simulink model "Flight_Model_2020b_11_28_2020"  (R2021a)
settings: Solver=ode45  StartTime=0.0  StopTime=100  RelTol=1e-3  EnableMultiTasking=on
model workspace (MAT data in the model file):
  bodyLength = 5
  brakesCd = 1
  brakesOn = 1
  dryCG = 1.9
  dryMass = 23
  finArea = 0.2
  finChordAngle = 0.5236
  finSpan = 0.4
  fullBrakesOn = 0
  gravity = 9.8067
  noseLength = 0.5
  propMass = 7.183
  refArea = 0.0182
  rocketCP = 1
  rocketDiam = 0.197
  targetAlt = 3048
  thrust = [0; 2638.366; 2528.97; 3063.078; 2426.009; 2548.275; 2599.755; 2554.71; 2644.801; 2638.366; 2561.145; 2606.19; 2638.366; 2638.366; 2580.45; 2496.795; 2335.919; 2213.653; 2129.998; 1653.805; 888.035; 630.634; 450.453; 289.577; 135.136; 25.74; 0]
  time = [0; 0.045; 0.067; 0.084; 0.124; 0.186; 0.231; 0.298; 0.371; 0.534; 0.979; 1.142; 2.002; 2.289; 2.761; 3.121; 3.436; 3.678; 3.79; 4.004; 4.415; 4.538; 4.656; 4.82; 5.005; 5.219; 5.371]
  totalImpulse = 10831
  vehicleCd = 0.8
  wetCG = 2.1
  wetMass = 30
undefined symbols (not defined in the file): Earth, WGS84, X, Y, Z
libraries: sm_lib x19, nesl_utility x10, aerolibasang x4, commchan3 x3, aerolibbdyn x2, aerolibwind2 x2, shared6dof x2, simulink x2, aerolibtransform2 x1, aerolibfltsims x1, aerolibatmos2 x1, aerolibconvert2 x1
(part 1 of 2)
settings Model: Creator=jacob  LastModifiedBy=alhus
settings SolverCC: AlgebraicLoopSolver=TrustRegion
settings DataIOCC: LimitDataPoints=on  SaveFormat=Array  ReturnWorkspaceOutputs=off
settings OptimizationCC: LifeSpan=inf
settings DebuggingCC: SFUnexpectedBacktrackingDiag=warning  SFNoUnconditionalDefaultTransitionDiag=warning  SFExecutionAtInitializationDiag=none  SFMachineParentedDataDiag=warning  ArithmeticOperatorsInVariantConditions=warning
settings HardwareCC: ProdBitPerPointer=32  ProdBitPerSizeT=32  ProdBitPerPtrDiffT=32  ProdLargestAtomicFloat=None  ProdIntDivRoundTo=Undefined  ProdEndianess=Unspecified  ProdWordSize=32  ProdHWDeviceType=32-bit Generic
settings ModelReferenceCC: PropagateSignalLabelsOutOfModel=off
settings SFSimCC: SimUseLocalCustomCode=off  CustomCodeUndefinedFunction=UseInterfaceOnly
settings RTWCC: RTWUseLocalCustomCode=off
settings CodeAppCC: StateflowObjectComments=on
settings GRTTargetCC: TargetLangStandard=C89/C90 (ANSI)
settings ConfigComp: CovMetricSettings=dw  CovSaveCumulativeToWorkspaceVar=on  CovSaveSingleToWorkspaceVar=on  CovExternalEMLEnable=off
settings SimscapeCC: SimscapeNormalizeSystem=off
settings ConfigurationSet: Description=SimMechanics 2G

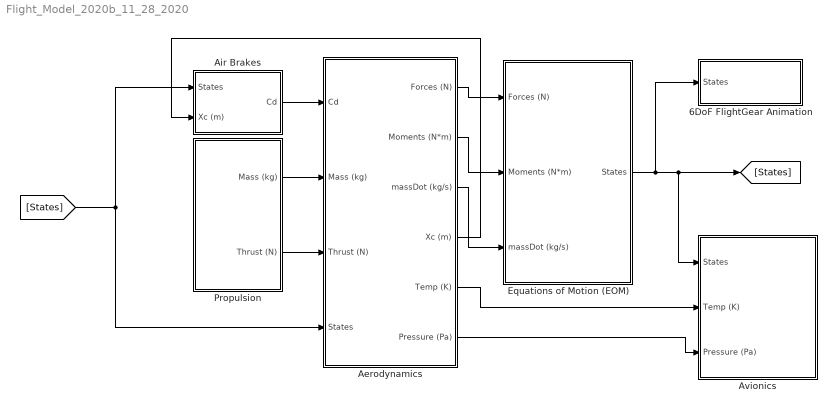
== system Flight_Model_2020b_11_28_2020 ==
  6DoF FlightGear Animation : Subsystem
  Aerodynamics : Subsystem
  Air Brakes : Subsystem
  Avionics : Subsystem
  Equations of Motion (EOM) : Subsystem
  Propulsion : Subsystem
  wires:
  Aerodynamics/1(Forces (N)) -> Equations of Motion (EOM)/1(Forces (N))
  Aerodynamics/2(Moments (N*m)) -> Equations of Motion (EOM)/2(Moments (N*m))
  Propulsion/1(Mass (kg)) -> Aerodynamics/2(Mass (kg))
  Propulsion/2(Thrust (N)) -> Aerodynamics/3(Thrust (N))
  Air Brakes/1("Cd ") -> Aerodynamics/1(Cd)
  Equations of Motion (EOM)/1(States) -> Avionics/1(States), [States], 6DoF FlightGear Animation/1(States)
  [States] -> Air Brakes/1(States), Aerodynamics/4(States)
  Aerodynamics/3(massDot (kg/s)) -> Equations of Motion (EOM)/3(massDot (kg/s))
  Aerodynamics/4(Xc (m)) -> Air Brakes/2(Xc (m))
  Aerodynamics/5(Temp (K)) -> Avionics/2(Temp (K))
  Aerodynamics/6(Pressure (Pa)) -> Avionics/3(Pressure (Pa))

== system Flight_Model_2020b_11_28_2020/6DoF FlightGear Animation ==
  States : Inport
  Bus Selector : BusSelector  OutputSignals=signal2,signal3
  Constant : Constant  Value=0
  Demux : Demux  Outputs=2
  Demux1 : Demux  Outputs=3
  Display : Display
  Display1 : Display
  Display2 : Display
  Flat Earth to LLA : aerolibtransform2/Flat Earth to LLA  units=Metric (MKS)  ptype=Earth (WGS84)  F=1/298.257223563  R=6378137  refPosPort=off  LL0=[0 10]  psi=0
  FlightGear Preconfigured 6DoF Animation : aerolibfltsims/FlightGear Preconfigured 6DoF Animation  xFlightGearVersion=v3.0  DestinationIpAddress=127.0.0.1  DestinationPort=5502  SampleTime=1/30  packetVersion=24
  Mux : Mux  Inputs=6
  wires:
  States/1 -> Bus Selector/1
  Constant/1 -> Flat Earth to LLA/2
  Mux/1 -> FlightGear Preconfigured 6DoF Animation/1
  Flat Earth to LLA/1 -> Demux/1
  Demux/1 -> Display1/1, Mux/2
  Demux/2 -> Display2/1, Mux/1
  Flat Earth to LLA/2 -> Display/1, Mux/3
  Demux1/2 -> Mux/5
  Demux1/3 -> Mux/6
  Demux1/1 -> Mux/4
  Bus Selector/1 -> Flat Earth to LLA/1  "<signal2>"
  Bus Selector/2 -> Demux1/1  "<signal3>"

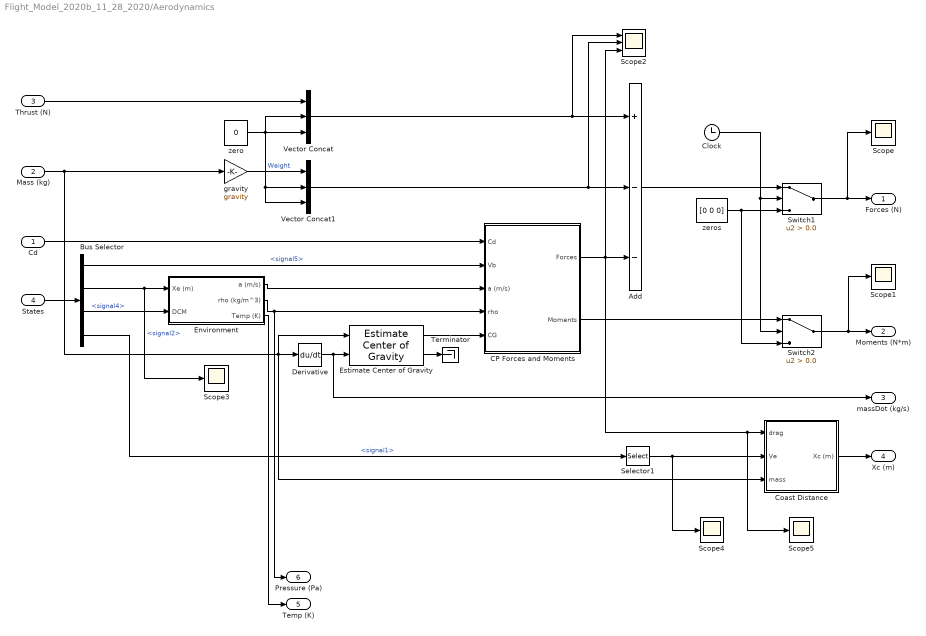
== system Flight_Model_2020b_11_28_2020/Aerodynamics ==
  Cd : Inport
  Mass (kg) : Inport  Port=2
  Thrust (N) : Inport  Port=3
  States : Inport  Port=4
  Add : Sum  Inputs=+--
  Bus Selector : BusSelector  OutputSignals=signal5,signal2,signal4,signal1
  CP Forces and Moments : Subsystem
  Clock : Clock
  Coast Distance : Subsystem
  Derivative : Derivative
  Environment : Subsystem
  Estimate Center of Gravity : aerolibbdyn/Estimate Center of Gravity  fmass=wetMass  emass=dryMass  fcg=[wetCG 0 0]'  ecg=[dryCG 0 0]'
      settings: SourceProductBaseCode=AE
  Scope{,1,3..5} (5 alike) : Scope
  Scope2 : Scope  NumInputPorts=3
  Selector1 : Selector  InputPortWidth=3  IndexOptions=Index vector (dialog)  Indices=1  OutputSizes=1
  Switch1 : Switch  Criteria=u2 > Threshold  Threshold=0.0
  Switch2 : Switch  Criteria=u2 > Threshold  Threshold=0.0
  Terminator : Terminator
  Vector Concat : Concatenate  NumInputs=3
  Vector Concat1 : Concatenate  NumInputs=3
  gravity : Gain  Gain=gravity
  "zero " : Constant  Value=0
  "zeros " : Constant  Value=[0 0 0]
  Forces (N) : Outport
  Moments (N*m) : Outport  Port=2
  massDot (kg/s) : Outport  Port=3
  Xc (m) : Outport  Port=4
  Temp (K) : Outport  Port=5
  Pressure (Pa) : Outport  Port=6
  wires:
  Mass (kg)/1 -> Coast Distance/3(mass), Estimate Center of Gravity/1, Derivative/1, gravity/1
  Derivative/1 -> Estimate Center of Gravity/2, massDot (kg/s)/1
  Estimate Center of Gravity/2 -> Terminator/1
  Estimate Center of Gravity/1 -> CP Forces and Moments/5(CG)
  Cd/1 -> CP Forces and Moments/1(Cd)
  Environment/2(rho (kg/m^3)) -> Pressure (Pa)/1, CP Forces and Moments/4(rho)
  Add/1 -> Switch1/1
  Switch1/1 -> Scope/1, Forces (N)/1
  "zeros "/1 -> Switch2/3, Switch1/3
  Clock/1 -> Switch2/2, Switch1/2
  Switch2/1 -> Scope1/1, Moments (N*m)/1
  States/1 -> Bus Selector/1
  Environment/1(a (m/s)) -> CP Forces and Moments/3(a (m/s))
  Bus Selector/1 -> CP Forces and Moments/2(Vb)  "<signal5>"
  Bus Selector/2 -> Environment/1(Xe (m)), Scope3/1  "<signal2>"
  Bus Selector/3 -> Environment/2(DCM)  "<signal4>"
  "zero "/1 -> Vector Concat/2, Vector Concat/3, Vector Concat1/2, Vector Concat1/3
  Thrust (N)/1 -> Vector Concat/1
  Vector Concat/1 -> Scope2/1, Add/1
  Vector Concat1/1 -> Scope2/2, Add/2
  CP Forces and Moments/2(Moments) -> Switch2/1
  gravity/1 -> Vector Concat1/1  "Weight"
  CP Forces and Moments/1(Forces) -> Scope5/1, Coast Distance/1(drag), Add/3, Scope2/3
  Bus Selector/4 -> Selector1/1  "<signal1>"
  Coast Distance/1(Xc (m)) -> Xc (m)/1
  Selector1/1 -> Coast Distance/2(Ve), Scope4/1
  Environment/3(Temp (K)) -> Temp (K)/1

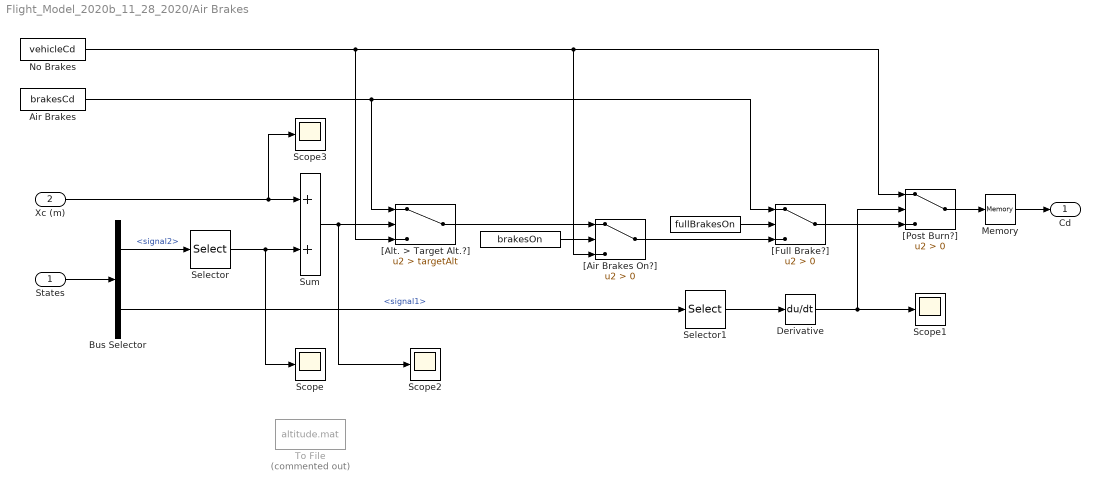
== system Flight_Model_2020b_11_28_2020/Air Brakes ==
  States : Inport
  Xc (m) : Inport  Port=2
  " " : Constant  Value=fullBrakesOn
  "  " : Constant  Value=brakesOn
  Air Brakes : Constant  Value=brakesCd
  Bus Selector : BusSelector  OutputSignals=signal2,signal1
  Derivative : Derivative
  Memory : Memory
  No Brakes : Constant  Value=vehicleCd
  Scope{,1..3} (4 alike) : Scope
  "Selector " : Selector  InputPortWidth=3  IndexOptions=Index vector (dialog)  Indices=1  OutputSizes=1
  Selector1 : Selector  InputPortWidth=3  IndexOptions=Index vector (dialog)  Indices=1  OutputSizes=1
  Sum : Sum
  To File : ToFile  Commented=on  Filename=altitude.mat  SaveFormat=Timeseries
  "[Air Brakes On?]" : Switch  Description=[Air Brakes On?]  Criteria=u2 > Threshold
  "[Alt. > Target Alt.?]" : Switch  Criteria=u2 > Threshold  Threshold=targetAlt
  "[Full Brake?]" : Switch  Criteria=u2 > Threshold
  "[Post Burn?]" : Switch  Criteria=u2 > Threshold
  "Cd " : Outport
  wires:
  Sum/1 -> Scope2/1, "[Alt. > Target Alt.?]"/2
  "[Post Burn?]"/1 -> Memory/1
  No Brakes/1 -> "[Alt. > Target Alt.?]"/3, "[Post Burn?]"/1, "[Air Brakes On?]"/3
  " "/1 -> "[Full Brake?]"/2
  Air Brakes/1 -> "[Alt. > Target Alt.?]"/1, "[Full Brake?]"/1
  "[Full Brake?]"/1 -> "[Post Burn?]"/3
  "Selector "/1 -> Scope/1, Sum/2
  "  "/1 -> "[Air Brakes On?]"/2
  "[Air Brakes On?]"/1 -> "[Full Brake?]"/3
  "[Alt. > Target Alt.?]"/1 -> "[Air Brakes On?]"/1
  States/1 -> Bus Selector/1
  Selector1/1 -> Derivative/1
  Derivative/1 -> "[Post Burn?]"/2, Scope1/1
  Bus Selector/1 -> "Selector "/1  "<signal2>"
  Xc (m)/1 -> Scope3/1, Sum/1
  Bus Selector/2 -> Selector1/1  "<signal1>"
  Memory/1 -> "Cd "/1

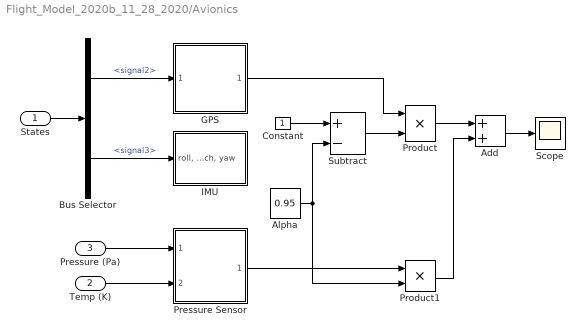
== system Flight_Model_2020b_11_28_2020/Avionics ==
  States : Inport
  Temp (K) : Inport  Port=2
  Pressure (Pa) : Inport  Port=3
  Add : Sum
  Alpha : Constant  Value=0.95
  Bus Selector : BusSelector  OutputSignals=signal2,signal3
  Constant : Constant
  GPS : Subsystem
  IMU : Subsystem
  Pressure Sensor : Subsystem
  Product : Product
  Product1 : Product
  Scope : Scope
  Subtract : Sum  Inputs=+-
  wires:
  States/1 -> Bus Selector/1
  Temp (K)/1 -> Pressure Sensor/2("Temp (K) ")
  Pressure (Pa)/1 -> Pressure Sensor/1(Pressure (Pa))
  Bus Selector/1 -> GPS/1(altitude)  "<signal2>"
  Bus Selector/2 -> IMU/1("roll, pitch, yaw")  "<signal3>"
  Constant/1 -> Subtract/1
  Alpha/1 -> Product1/2, Subtract/2
  Subtract/1 -> Product/2
  GPS/1(GPS Alt) -> Product/1
  Product/1 -> Add/1
  Pressure Sensor/1(BMP Alt) -> Product1/1
  Product1/1 -> Add/2
  Add/1 -> Scope/1

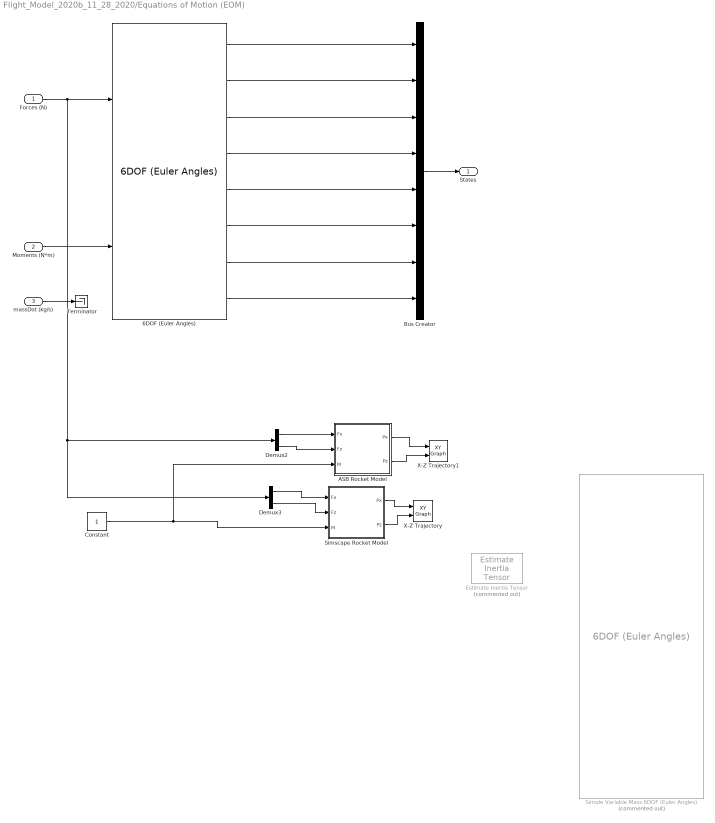
== system Flight_Model_2020b_11_28_2020/Equations of Motion (EOM) ==
  Forces (N) : Inport
  Moments (N*m) : Inport  Port=2
  massDot (kg/s) : Inport  Port=3
  6DOF (Euler Angles) : shared6dof/6DOF (Euler Angles)  units=Metric (MKS)  mtype=Fixed  rep=Euler Angles  xme_0=[0 0 0]  Vm_0=[0 0 0]  eul_0=[0 0 0]  pm_0=[0, 0, 0]  mass_0=30  mass_e=0.5  mass_f=2.0  inertia=eye(3)  inertia_e=eye(3)  inertia_f=2*eye(3)  k_quat=1.0  vre_flag=on  abi_flag=off  aMode=aMode  xme_statename=''  Vm_statename=''  eul_statename=''  quat_statename=''  pm_statename=''  mass_statename=''
      settings: SourceProductBaseCode=AE,PW,DR,MT,UV,VE
  ASB Rocket Model : Subsystem  VariantControl=VSS_MODE == 0
  Bus Creator : BusCreator  Inputs=8
  Constant : Constant
  Demux2 : Demux  Outputs=3
  Demux3 : Demux  Outputs=3
  Estimate Inertia Tensor : shareddyn/Estimate Inertia Tensor  Commented=on  fmass=2  emass=1  fI=eye(3)  eI=eye(3)/2  aMode=aMode
      settings: SourceProductBaseCode=AE,PW,DR,MT,UV,VE
  Simple Variable Mass 6DOF (Euler Angles) : shared6dof/6DOF (Euler Angles)  Commented=on  units=Metric (MKS)  mtype=Simple Variable  rep=Euler Angles  xme_0=[0 0 0]  Vm_0=[0 0 0]  eul_0=[0 0 0]  pm_0=[0 0 0]  mass_0=1.0  mass_e=0.5  mass_f=2.0  inertia=eye(3)  inertia_e=eye(3)  inertia_f=2*eye(3)  k_quat=1.0  vre_flag=off  abi_flag=off  aMode=aMode  xme_statename=''  Vm_statename=''  eul_statename=''  quat_statename=''  pm_statename=''  mass_statename=''
      settings: SourceProductBaseCode=AE,PW,DR,MT,UV,VE
  Simscape Rocket Model : Subsystem  VariantControl=VSS_MODE == 1
  Terminator : Terminator
  X-Z Trajectory : simulink/Sinks/XY Graph  xmin=-20  xmax=20  ymin=0  ymax=100  st=-1
  X-Z Trajectory1 : simulink/Sinks/XY Graph  xmin=-20  xmax=20  ymin=0  ymax=100  st=-1
  States : Outport
  wires:
  6DOF (Euler Angles)/2 -> Bus Creator/2
  6DOF (Euler Angles)/1 -> Bus Creator/1
  Bus Creator/1 -> States/1
  6DOF (Euler Angles)/3 -> Bus Creator/3
  6DOF (Euler Angles)/4 -> Bus Creator/4
  6DOF (Euler Angles)/5 -> Bus Creator/5
  6DOF (Euler Angles)/6 -> Bus Creator/6
  6DOF (Euler Angles)/7 -> Bus Creator/7
  6DOF (Euler Angles)/8 -> Bus Creator/8
  massDot (kg/s)/1 -> Terminator/1
  Demux3/1 -> Simscape Rocket Model/1(Fx)
  Demux2/1 -> ASB Rocket Model/1(Fx)
  ASB Rocket Model/2(Pz) -> X-Z Trajectory1/2
  Demux2/3 -> ASB Rocket Model/2(Fz)
  Moments (N*m)/1 -> 6DOF (Euler Angles)/2
  Simscape Rocket Model/1(Px) -> X-Z Trajectory/1
  Demux3/3 -> Simscape Rocket Model/2(Fz)
  ASB Rocket Model/1(Px) -> X-Z Trajectory1/1
  Simscape Rocket Model/2(Pz) -> X-Z Trajectory/2
  Forces (N)/1 -> Demux3/1, Demux2/1, 6DOF (Euler Angles)/1
  Constant/1 -> ASB Rocket Model/3(M), Simscape Rocket Model/3(M)

== system Flight_Model_2020b_11_28_2020/Propulsion ==
  Clock : Clock
  Divide : Product  Inputs=*/
  Integrator : Integrator
  Product : Product
  Propellant Mass : Constant  Value=propMass
  Rocket Mass : Constant  Value=wetMass
  Subtract : Sum  Inputs=+-
  Thrust Curve Table : Lookup_n-D  NumberOfTableDimensions=1  BreakpointsForDimension1=time  Table=thrust  ExtrapMethod=Clip  InternalRulePriority=Speed  RndMeth=Simplest  InputSameDT=on
  Total Impulse : Constant  Value=totalImpulse
  Mass (kg) : Outport
  Thrust (N) : Outport  Port=2
  wires:
  Total Impulse/1 -> Divide/2
  Integrator/1 -> Divide/1
  Clock/1 -> Thrust Curve Table/1
  Propellant Mass/1 -> Product/1
  Product/1 -> Subtract/2  "Burnt Propellant Mass"
  Rocket Mass/1 -> Subtract/1
  Subtract/1 -> Mass (kg)/1
  Thrust Curve Table/1 -> Thrust (N)/1, Integrator/1
  Divide/1 -> Product/2  "Percentage of Impulse"

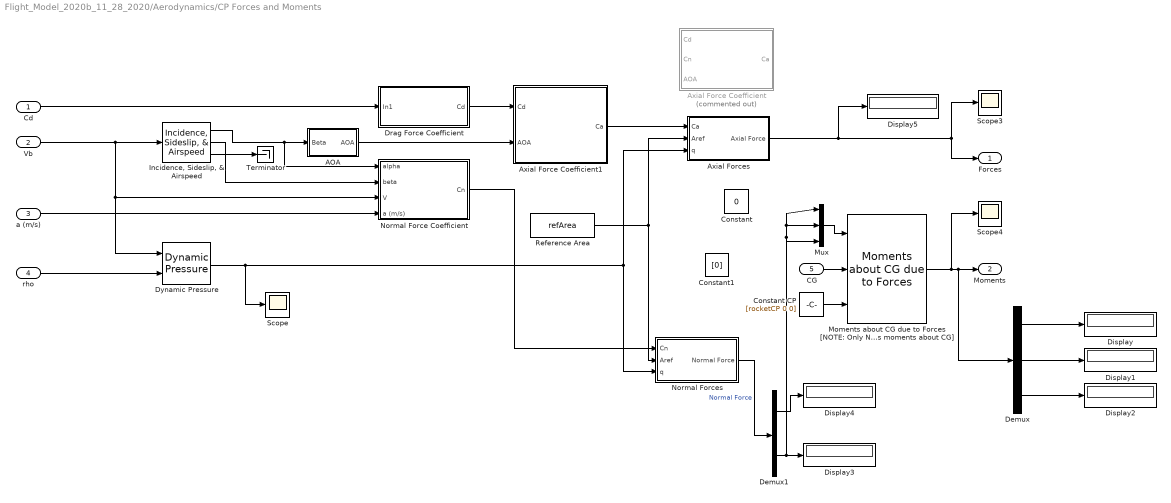
== system Flight_Model_2020b_11_28_2020/Aerodynamics/CP Forces and Moments ==
  Cd : Inport
  Vb : Inport  Port=2
  a (m/s) : Inport  Port=3
  rho : Inport  Port=4
  CG : Inport  Port=5
  AOA : Subsystem
  Axial Force Coefficient : Subsystem  Commented=on
  Axial Force Coefficient1 : Subsystem
  Axial Forces : Subsystem
  Constant : Constant  Value=0
  Constant CP : Constant  Value=[rocketCP 0 0]
  Constant1 : Constant  Value=[0]
  Demux : Demux  Outputs=3
  Demux1 : Demux  Outputs=2
  Display{,1..5} (6 alike) : Display
  Drag Force Coefficient : Subsystem
  Dynamic Pressure : aerolibasang/Dynamic Pressure
  "Incidence, Sideslip, & Airspeed" : aerolibasang/Incidence, Sideslip, & Airspeed
  Moments about CG due to Forces [NOTE: Only Normal Force applys moments about CG] : aerolibbdyn/Moments about CG  due to Forces
      settings: SourceProductBaseCode=AE
  Mux : Mux  Inputs=3
  Normal Force Coefficient : Subsystem
  Normal Forces : Subsystem
  Reference Area : Constant  Value=refArea
  Scope : Scope
  Scope3 : Scope
  Scope4 : Scope
  Terminator : Terminator
  Forces : Outport
  Moments : Outport  Port=2
  wires:
  CG/1 -> Moments about CG due to Forces [NOTE: Only Normal Force applys moments about CG]/2
  Vb/1 -> Dynamic Pressure/1, Normal Force Coefficient/3(V), "Incidence, Sideslip, & Airspeed"/1
  Drag Force Coefficient/1(Cd) -> Axial Force Coefficient1/1(Cd)
  Axial Force Coefficient1/1(Ca) -> Axial Forces/1(Ca)
  Axial Forces/1(Axial Force) -> Display5/1, Forces/1, Scope3/1
  rho/1 -> Dynamic Pressure/2
  a (m/s)/1 -> Normal Force Coefficient/4(a (m/s))
  Dynamic Pressure/1 -> Scope/1, Normal Forces/3("q "), Axial Forces/3("q ")
  AOA/1(AOA) -> Axial Force Coefficient1/2(AOA)
  Cd/1 -> Drag Force Coefficient/1(In1)
  Reference Area/1 -> Normal Forces/2(Aref), Axial Forces/2(Aref)
  Constant CP/1 -> Moments about CG due to Forces [NOTE: Only Normal Force applys moments about CG]/3
  Moments about CG due to Forces [NOTE: Only Normal Force applys moments about CG]/1 -> Scope4/1, Demux/1, Moments/1
  "Incidence, Sideslip, & Airspeed"/1 -> Normal Force Coefficient/1(alpha), AOA/1(Beta)
  "Incidence, Sideslip, & Airspeed"/2 -> Normal Force Coefficient/2(beta)
  "Incidence, Sideslip, & Airspeed"/3 -> Terminator/1
  Demux/1 -> Display/1
  Demux/2 -> Display1/1
  Demux/3 -> Display2/1
  Mux/1 -> Moments about CG due to Forces [NOTE: Only Normal Force applys moments about CG]/1
  Normal Force Coefficient/1(Cn) -> Normal Forces/1(Cn)
  Demux1/2 -> Mux/1, Mux/2, Mux/3, Display3/1
  Normal Forces/1(Normal Force) -> Demux1/1  "Normal Force"
  Demux1/1 -> Display4/1

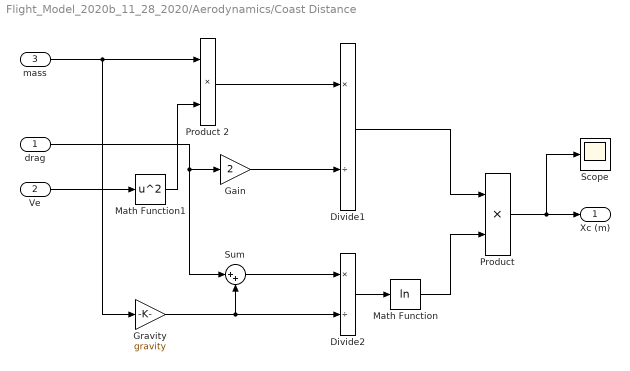
== system Flight_Model_2020b_11_28_2020/Aerodynamics/Coast Distance ==
  drag : Inport
  Ve : Inport  Port=2
  mass : Inport  Port=3
  Divide1 : Product  Inputs=*/
  Divide2 : Product  Inputs=*/
  Gain : Gain  Gain=2
  Gravity : Gain  Gain=gravity
  Math Function : Math  Operator=log  SignedPower=on  SaturateOnIntegerOverflow=on
  Math Function1 : Math  Operator=square  SignedPower=on  SaturateOnIntegerOverflow=on
  Product : Product
  Product 2 : Product  Inputs=**
  Scope : Scope
  Sum : Sum  Inputs=|++
  Xc (m) : Outport
  wires:
  Math Function/1 -> Product/2
  mass/1 -> Gravity/1, Product 2/1
  Divide1/1 -> Product/1
  drag/1 -> Gain/1, Sum/1
  Divide2/1 -> Math Function/1
  Product/1 -> Xc (m)/1, Scope/1
  Sum/1 -> Divide2/1
  Gravity/1 -> Sum/2, Divide2/2
  Ve/1 -> Math Function1/1
  Math Function1/1 -> Product 2/2
  Product 2/1 -> Divide1/1
  Gain/1 -> Divide1/2

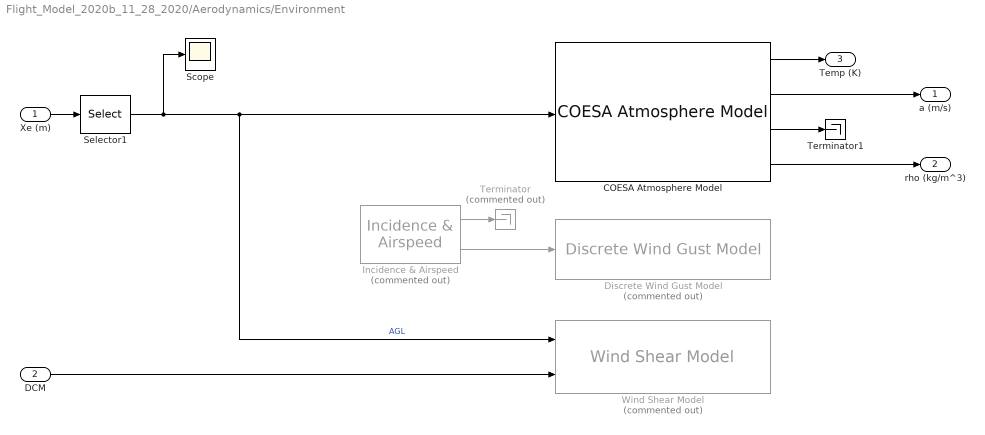
== system Flight_Model_2020b_11_28_2020/Aerodynamics/Environment ==
  Xe (m) : Inport
  DCM : Inport  Port=2
  COESA Atmosphere Model : aerolibatmos2/COESA Atmosphere Model  units=Metric (MKS)  spec=1976 COESA-extended U.S. Standard Atmosphere  model=Profile  profile_var=High temperature  profile_percent=1%  profile_alt=5 km (16404 ft)  envelope_var=High temperature  envelope_percent=1%  action=Warning
  Discrete Wind Gust Model : aerolibwind2/Discrete Wind Gust Model  Commented=on  units=Metric (MKS)  Gx=on  Gy=on  Gz=on  t_0=5  d_m=[120 120 80]  v_m=[3.5 3.5 3.0]
  Incidence & Airspeed : aerolibasang/Incidence  & Airspeed  Commented=on
      settings: SourceProductBaseCode=AE
  Scope : Scope
  Selector1 : Selector  InputPortWidth=3  IndexOptions=Index vector (dialog)  Indices=3  OutputSizes=1
  Terminator : Terminator  Commented=on
  Terminator1 : Terminator
  Wind Shear Model : aerolibwind2/Wind Shear Model  Commented=on  units=Metric (MKS)  phase=Category C - Terminal Flight Phase  W_20=15  Wdeg=0
  a (m/s) : Outport
  rho (kg/m^3) : Outport  Port=2
  Temp (K) : Outport  Port=3
  wires:
  Incidence & Airspeed/2 -> Discrete Wind Gust Model/1
  Incidence & Airspeed/1 -> Terminator/1
  Xe (m)/1 -> Selector1/1
  DCM/1 -> Wind Shear Model/2
  Selector1/1 -> Wind Shear Model/1, COESA Atmosphere Model/1, Scope/1  "AGL"
  COESA Atmosphere Model/2 -> a (m/s)/1
  COESA Atmosphere Model/4 -> rho (kg/m^3)/1
  COESA Atmosphere Model/1 -> Temp (K)/1
  COESA Atmosphere Model/3 -> Terminator1/1

== system Flight_Model_2020b_11_28_2020/Avionics/GPS ==
  altitude : Inport
  AWGN Channel : commchan3/AWGN Channel  InputProcessing=Columns as channels (frame based)  seed=67  noiseMode=Variance from port  EbNodB=10  EsNodB=10  SNRdB=10  bitsPerSym=1  Ps=1  Tsym=1  variance=1
  Add : Sum
  Constant : Constant  Value=3
  Gain : Gain  Gain=3
  Scope : Scope
  GPS Alt : Outport
  wires:
  altitude/1 -> Gain/1, Add/1
  Add/1 -> AWGN Channel/1
  Constant/1 -> AWGN Channel/2
  AWGN Channel/1 -> GPS Alt/1, Scope/1
  Gain/1 -> Add/2

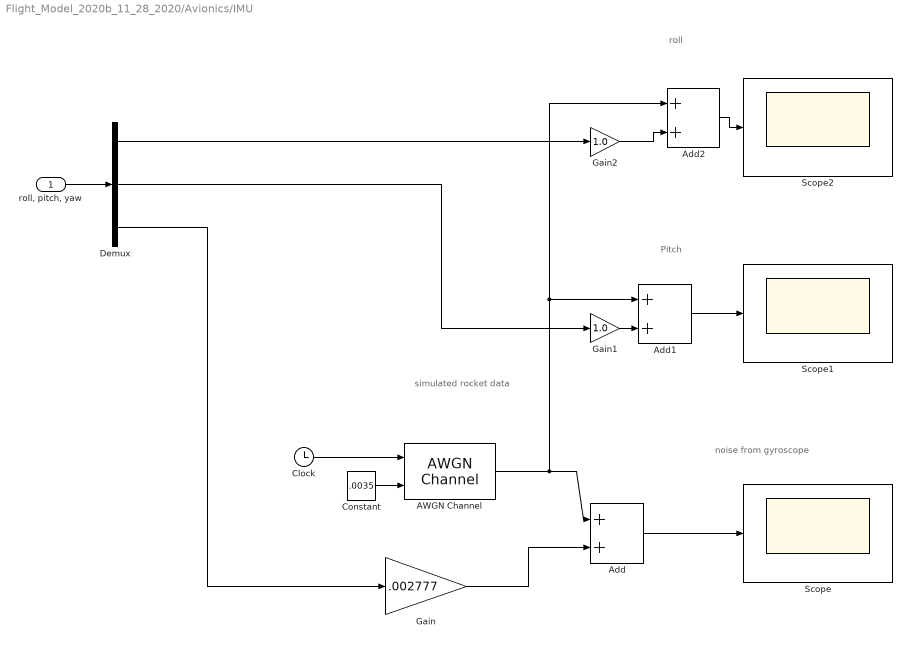
== system Flight_Model_2020b_11_28_2020/Avionics/IMU ==
  note: noise from gyroscope
  note: simulated rocket
      | data
  note: roll
  note: Pitch
  "roll, pitch, yaw" : Inport
  AWGN Channel : commchan3/AWGN Channel  InputProcessing=Columns as channels (frame based)  seed=67  noiseMode=Variance from port  EbNodB=10  EsNodB=10  SNRdB=10  bitsPerSym=1  Ps=1  Tsym=1  variance=1
  Add : Sum
  Add1 : Sum
  Add2 : Sum
  Clock : Clock
  Constant : Constant  Value=.0035
  Demux : Demux  Outputs=3
  Gain : Gain  Gain=.002777
  Gain1 : Gain  Gain=1.0
  Gain2 : Gain  Gain=1.0
  Scope : Scope
  Scope1 : Scope
  Scope2 : Scope
  wires:
  Constant/1 -> AWGN Channel/2
  Gain/1 -> Add/2
  Add/1 -> Scope/1
  Gain2/1 -> Add2/2
  AWGN Channel/1 -> Add1/1, Add2/1, Add/1
  Add1/1 -> Scope1/1
  Add2/1 -> Scope2/1
  Gain1/1 -> Add1/2
  "roll, pitch, yaw"/1 -> Demux/1
  Demux/1 -> Gain2/1
  Demux/2 -> Gain1/1
  Demux/3 -> Gain/1
  Clock/1 -> AWGN Channel/1

== system Flight_Model_2020b_11_28_2020/Avionics/Pressure Sensor ==
  Pressure (Pa) : Inport
  "Temp (K) " : Inport  Port=2
  AWGN Channel : commchan3/AWGN Channel  InputProcessing=Columns as channels (frame based)  seed=67  noiseMode=Variance from port  EbNodB=10  EsNodB=10  SNRdB=10  bitsPerSym=1  Ps=1  Tsym=1  variance=1
  Add : Sum
  Constant : Constant  Value=.5
  Gain : Gain
  Pa to hPa : Gain  Gain=0.01
  Pressure to Altitude : Subsystem
  Scope : Scope
  Temperature Conversion : aerolibconvert2/Temperature Conversion  IU=K  OU=C
      settings: SourceProductBaseCode=AE
  BMP Alt : Outport
  wires:
  Pa to hPa/1 -> Gain/1, Add/1
  Gain/1 -> Add/2
  Constant/1 -> AWGN Channel/2
  Add/1 -> Pressure to Altitude/1(Atmostpheric Pressure)
  AWGN Channel/1 -> BMP Alt/1, Scope/1
  Pressure to Altitude/1(Altitude) -> AWGN Channel/1
  Pressure (Pa)/1 -> Pa to hPa/1
  "Temp (K) "/1 -> Temperature Conversion/1
  Temperature Conversion/1 -> Pressure to Altitude/2("Temp (C) ")

== system Flight_Model_2020b_11_28_2020/Equations of Motion (EOM)/ASB Rocket Model ==
  Fx : Inport
  Fz : Inport  Port=2
  M : Inport  Port=3
  Demux : Demux  Outputs=2
  Gain1 : Gain  Gain=-1
  Rocket Model : shared3dof/3DOF (Body Axes)  units=Metric (MKS)  mtype=Fixed  v_ini=0  theta_ini=0  alpha_ini=0  pos_ini=[0 0]  q_ini=0  mass=0.8  mass_e=0.5  mass_f=3.0  Iyy=1  Iyy_e=0.5  Iyy_f=3.0  g_in=Internal  g=9.81  vre_flag=on  abi_flag=off  aMode=0  vel_statename=''  theta_statename=''  pos_statename=''  q_statename=''  mass_statename=''
      settings: SourceProductBaseCode=AE,PW,DR,MT,UV,VE
  Terminator{1..5} (5 alike) : Terminator
  Px : Outport
  Pz : Outport  Port=2
  wires:
  Rocket Model/2 -> Terminator2/1
  Rocket Model/4 -> Demux/1
  Demux/1 -> Px/1
  Rocket Model/6 -> Terminator5/1
  Rocket Model/1 -> Terminator1/1
  Demux/2 -> Gain1/1
  Fz/1 -> Rocket Model/2
  Rocket Model/5 -> Terminator4/1
  Fx/1 -> Rocket Model/1
  M/1 -> Rocket Model/3
  Rocket Model/3 -> Terminator3/1
  Gain1/1 -> Pz/1  "Pz"

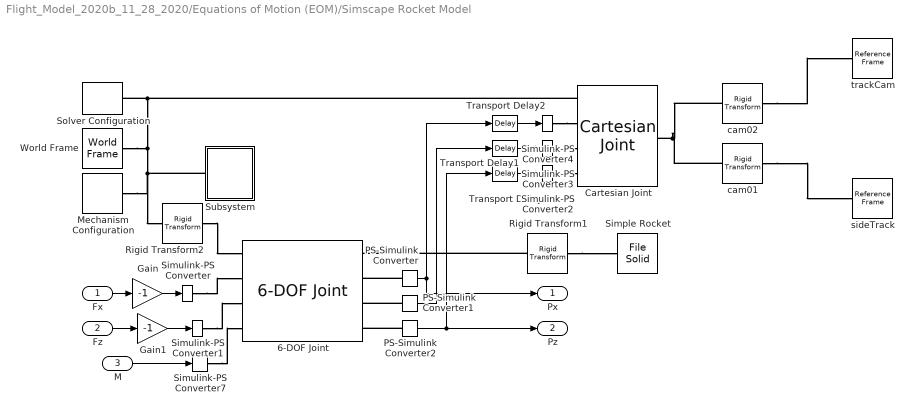
== system Flight_Model_2020b_11_28_2020/Equations of Motion (EOM)/Simscape Rocket Model ==
  Fx : Inport
  Fz : Inport  Port=2
  M : Inport  Port=3
  6-DOF Joint : sm_lib/Joints/6-DOF Joint  JointMode=Normal  SenseConstraintForce=off  SenseConstraintForceX=off  SenseConstraintForceY=off  SenseConstraintForceZ=off  SenseConstraintTorque=off  SenseConstraintTorqueX=off  SenseConstraintTorqueY=off  SenseConstraintTorqueZ=off  SenseTotalForce=off  SenseTotalForceX=off  SenseTotalForceY=off  SenseTotalForceZ=off  SenseTotalTorque=off  SenseTotalTorqueX=off  SenseTotalTorqueY=off  SenseTotalTorqueZ=off  CompositeWrenchDir=FollowerOnBase  CompositeWrenchFrame=BaseFrame  PxEquilibriumPosition=0  PxEquilibriumPositionUnits=m  PxSpringStiffness=0  PxSpringStiffnessUnits=N/m  PxDampingCoefficient=0  PxDampingCoefficientUnits=N/(m/s)  PxTorqueActuationMode=InputTorque  PxMotionActuationMode=ComputedMotion  PxSensePosition=on  PxSenseVelocity=off  PxSenseAcceleration=off  PxSenseTorqueForce=off  PxSenseLowerLimitTorqueForce=off  PxSenseUpperLimitTorqueForce=off  PxLowerLimitSpecify=off  PxLowerLimitBound=-1  PxLowerLimitBoundUnits=m  PxLowerLimitStiffness=1e6  PxLowerLimitStiffnessUnits=N/m  PxLowerLimitDamping=1e3  PxLowerLimitDampingUnits=N/(m/s)  PxLowerLimitTransitionRegionWidth=1e-4  PxLowerLimitTransitionRegionWidthUnits=m  PxUpperLimitSpecify=off  PxUpperLimitBound=1  PxUpperLimitBoundUnits=m  PxUpperLimitStiffness=1e6  PxUpperLimitStiffnessUnits=N/m  PxUpperLimitDamping=1e3  PxUpperLimitDampingUnits=N/(m/s)  PxUpperLimitTransitionRegionWidth=1e-4  PxUpperLimitTransitionRegionWidthUnits=m  PxPositionTargetSpecify=off  PxPositionTargetPriority=High  PxPositionTargetValue=0  PxPositionTargetValueUnits=m  PxVelocityTargetSpecify=off  PxVelocityTargetPriority=High  PxVelocityTargetValue=0  PxVelocityTargetValueUnits=m/s  PyEquilibriumPosition=0  PyEquilibriumPositionUnits=m  PySpringStiffness=0  PySpringStiffnessUnits=N/m  PyDampingCoefficient=0  PyDampingCoefficientUnits=N/(m/s)  PyTorqueActuationMode=NoTorque  PyMotionActuationMode=ComputedMotion  PySensePosition=on  PySenseVelocity=off  PySenseAcceleration=off  PySenseTorqueForce=off  PySenseLowerLimitTorqueForce=off  PySenseUpperLimitTorqueForce=off  PyLowerLimitSpecify=off  PyLowerLimitBound=-1  PyLowerLimitBoundUnits=m  PyLowerLimitStiffness=1e6  PyLowerLimitStiffnessUnits=N/m  PyLowerLimitDamping=1e3  PyLowerLimitDampingUnits=N/(m/s)  PyLowerLimitTransitionRegionWidth=1e-4  PyLowerLimitTransitionRegionWidthUnits=m  PyUpperLimitSpecify=off  PyUpperLimitBound=1  PyUpperLimitBoundUnits=m  PyUpperLimitStiffness=1e6  PyUpperLimitStiffnessUnits=N/m  PyUpperLimitDamping=1e3  PyUpperLimitDampingUnits=N/(m/s)  PyUpperLimitTransitionRegionWidth=1e-4  PyUpperLimitTransitionRegionWidthUnits=m  PyPositionTargetSpecify=off  PyPositionTargetPriority=High  PyPositionTargetValue=0  PyPositionTargetValueUnits=m  PyVelocityTargetSpecify=off  PyVelocityTargetPriority=High  PyVelocityTargetValue=0  PyVelocityTargetValueUnits=m/s  PzEquilibriumPosition=0  PzEquilibriumPositionUnits=m  PzSpringStiffness=0  PzSpringStiffnessUnits=N/m  PzDampingCoefficient=0  PzDampingCoefficientUnits=N/(m/s)  PzTorqueActuationMode=InputTorque  PzMotionActuationMode=ComputedMotion  PzSensePosition=on  PzSenseVelocity=off  PzSenseAcceleration=off  PzSenseTorqueForce=off  PzSenseLowerLimitTorqueForce=off  PzSenseUpperLimitTorqueForce=off  PzLowerLimitSpecify=off  PzLowerLimitBound=-1  PzLowerLimitBoundUnits=m  PzLowerLimitStiffness=1e6  PzLowerLimitStiffnessUnits=N/m  PzLowerLimitDamping=1e3  PzLowerLimitDampingUnits=N/(m/s)  PzLowerLimitTransitionRegionWidth=1e-4  PzLowerLimitTransitionRegionWidthUnits=m  PzUpperLimitSpecify=off  PzUpperLimitBound=1  PzUpperLimitBoundUnits=m  PzUpperLimitStiffness=1e6  PzUpperLimitStiffnessUnits=N/m  PzUpperLimitDamping=1e3  PzUpperLimitDampingUnits=N/(m/s)  PzUpperLimitTransitionRegionWidth=1e-4  PzUpperLimitTransitionRegionWidthUnits=m  PzPositionTargetSpecify=off  PzPositionTargetPriority=High  PzPositionTargetValue=1  PzPositionTargetValueUnits=m  PzVelocityTargetSpecify=off  PzVelocityTargetPriority=High  PzVelocityTargetValue=0  PzVelocityTargetValueUnits=m/s  SphDefPosRotationMethod=None  SphDefPosRotationAngleUnits=deg  SphDefPosRotationStandardAxis=+Z  SphDefPosRotationAngle=0.0  SphDefPosRotationArbitraryAxis=[0 0 1]  SphDefPosFollAlignAxisA=+X  SphDefPosBaseAlignAxisA=+Y  SphDefPosFollAlignAxisB=+Y  SphDefPosBaseAlignAxisB=+Z  SphDefPosRotationSequenceAxes=FollowerAxes  SphDefPosRotationSequence=XYX  SphDefPosRotationSequenceAngles=[0 0 0]  SphDefPosRotationSequenceAnglesUnits=deg  SphDefPosRotationMatrix=[1 0 0; 0 1 0; 0 0 1]  SphEqPosRotationMethod=None  SphEqPosRotationAngleUnits=deg  SphEqPosRotationStandardAxis=+Z  SphEqPosRotationAngle=0.0  SphEqPosRotationArbitraryAxis=[0 0 1]  SphEqPosFollAlignAxisA=+X  SphEqPosBaseAlignAxisA=+Y  SphEqPosFollAlignAxisB=+Y  SphEqPosBaseAlignAxisB=+Z  SphEqPosRotationSequenceAxes=FollowerAxes  SphEqPosRotationSequence=XYX  SphEqPosRotationSequenceAngles=[0 0 0]  SphEqPosRotationSequenceAnglesUnits=deg  SphEqPosRotationMatrix=[1 0 0; 0 1 0; 0 0 1]  SphSpringStiffness=0  SphSpringStiffnessUnits=N*m/deg  SphDampingCoefficient=0  SphDampingCoefficientUnits=N*m/(deg/s)  SphActuateTorqueX=off  SphActuateTorqueY=on  SphActuateTorqueZ=off  SphActuateTorque=off  SphTorqueActuationMode=InputTorque  SphMotionActuationMode=ComputedMotion  SphActuationFrame=BaseFrame  SphSensePosition=off  SphSenseVelocityX=off  SphSenseVelocityY=off  SphSenseVelocityZ=off  SphSenseVelocity=off  SphSenseAccelerationX=off  SphSenseAccelerationY=off  SphSenseAccelerationZ=off  SphSenseAcceleration=off  SphSenseTorqueX=off  SphSenseTorqueY=off  SphSenseTorqueZ=off  SphSenseTorqueForce=off  SphSenseLowerLimitTorqueMag=off  SphSenseUpperLimitTorqueMag=off  SphSensingFrame=BaseFrame  SphLowerLimitSpecify=off  SphLowerLimitBound=15  SphLowerLimitBoundUnits=deg  SphLowerLimitStiffness=1e4  SphLowerLimitStiffnessUnits=N*m/deg  SphLowerLimitDamping=10  SphLowerLimitDampingUnits=N*m/(deg/s)  SphLowerLimitTransitionRegionWidth=0.1  SphLowerLimitTransitionRegionWidthUnits=deg  SphUpperLimitSpecify=off  SphUpperLimitBound=45  SphUpperLimitBoundUnits=deg  SphUpperLimitStiffness=1e4  SphUpperLimitStiffnessUnits=N*m/deg  SphUpperLimitDamping=10  SphUpperLimitDampingUnits=N*m/(deg/s)  SphUpperLimitTransitionRegionWidth=0.1  SphUpperLimitTransitionRegionWidthUnits=deg  SphPositionTargetRotationMethod=None  SphPositionTargetRotationAngleUnits=deg  SphPositionTargetRotationStandardAxis=+Z  SphPositionTargetRotationAngle=0.0  SphPositionTargetRotationArbitraryAxis=[0 0 1]  SphPositionTargetFollAlignAxisA=+X  SphPositionTargetBaseAlignAxisA=+Y  SphPositionTargetFollAlignAxisB=+Y  SphPositionTargetBaseAlignAxisB=+Z  SphPositionTargetRotationSequenceAxes=FollowerAxes  SphPositionTargetRotationSequence=XYX  SphPositionTargetRotationSequenceAngles=[0 0 0]  SphPositionTargetRotationSequenceAnglesUnits=deg  SphPositionTargetRotationMatrix=[1 0 0; 0 1 0; 0 0 1]  SphPositionTargetSpecify=off  SphPositionTargetPriority=High  SphVelocityTargetValue=[0 0 0]  SphVelocityTargetValueUnits=deg/s  SphVelocityTargetSpecify=off  SphVelocityTargetPriority=High  SphVelocityTargetInFollowerFrame=on
  Cartesian Joint : sm_lib/Joints/Cartesian Joint  JointMode=Normal  SenseConstraintForce=off  SenseConstraintForceX=off  SenseConstraintForceY=off  SenseConstraintForceZ=off  SenseConstraintTorque=off  SenseConstraintTorqueX=off  SenseConstraintTorqueY=off  SenseConstraintTorqueZ=off  SenseTotalForce=off  SenseTotalForceX=off  SenseTotalForceY=off  SenseTotalForceZ=off  SenseTotalTorque=off  SenseTotalTorqueX=off  SenseTotalTorqueY=off  SenseTotalTorqueZ=off  CompositeWrenchDir=FollowerOnBase  CompositeWrenchFrame=BaseFrame  PxEquilibriumPosition=0  PxEquilibriumPositionUnits=m  PxSpringStiffness=0  PxSpringStiffnessUnits=N/m  PxDampingCoefficient=0  PxDampingCoefficientUnits=N/(m/s)  PxTorqueActuationMode=ComputedTorque  PxMotionActuationMode=InputMotion  PxSensePosition=off  PxSenseVelocity=off  PxSenseAcceleration=off  PxSenseTorqueForce=off  PxSenseLowerLimitTorqueForce=off  PxSenseUpperLimitTorqueForce=off  PxLowerLimitSpecify=off  PxLowerLimitBound=-1  PxLowerLimitBoundUnits=m  PxLowerLimitStiffness=1e6  PxLowerLimitStiffnessUnits=N/m  PxLowerLimitDamping=1e3  PxLowerLimitDampingUnits=N/(m/s)  PxLowerLimitTransitionRegionWidth=1e-4  PxLowerLimitTransitionRegionWidthUnits=m  PxUpperLimitSpecify=off  PxUpperLimitBound=1  PxUpperLimitBoundUnits=m  PxUpperLimitStiffness=1e6  PxUpperLimitStiffnessUnits=N/m  PxUpperLimitDamping=1e3  PxUpperLimitDampingUnits=N/(m/s)  PxUpperLimitTransitionRegionWidth=1e-4  PxUpperLimitTransitionRegionWidthUnits=m  PxPositionTargetSpecify=off  PxPositionTargetPriority=High  PxPositionTargetValue=0  PxPositionTargetValueUnits=m  PxVelocityTargetSpecify=off  PxVelocityTargetPriority=High  PxVelocityTargetValue=0  PxVelocityTargetValueUnits=m/s  PyEquilibriumPosition=0  PyEquilibriumPositionUnits=m  PySpringStiffness=0  PySpringStiffnessUnits=N/m  PyDampingCoefficient=0  PyDampingCoefficientUnits=N/(m/s)  PyTorqueActuationMode=ComputedTorque  PyMotionActuationMode=InputMotion  PySensePosition=off  PySenseVelocity=off  PySenseAcceleration=off  PySenseTorqueForce=off  PySenseLowerLimitTorqueForce=off  PySenseUpperLimitTorqueForce=off  PyLowerLimitSpecify=off  PyLowerLimitBound=-1  PyLowerLimitBoundUnits=m  PyLowerLimitStiffness=1e6  PyLowerLimitStiffnessUnits=N/m  PyLowerLimitDamping=1e3  PyLowerLimitDampingUnits=N/(m/s)  PyLowerLimitTransitionRegionWidth=1e-4  PyLowerLimitTransitionRegionWidthUnits=m  PyUpperLimitSpecify=off  PyUpperLimitBound=1  PyUpperLimitBoundUnits=m  PyUpperLimitStiffness=1e6  PyUpperLimitStiffnessUnits=N/m  PyUpperLimitDamping=1e3  PyUpperLimitDampingUnits=N/(m/s)  PyUpperLimitTransitionRegionWidth=1e-4  PyUpperLimitTransitionRegionWidthUnits=m  PyPositionTargetSpecify=off  PyPositionTargetPriority=High  PyPositionTargetValue=0  PyPositionTargetValueUnits=m  PyVelocityTargetSpecify=off  PyVelocityTargetPriority=High  PyVelocityTargetValue=0  PyVelocityTargetValueUnits=m/s  PzEquilibriumPosition=0  PzEquilibriumPositionUnits=m  PzSpringStiffness=0  PzSpringStiffnessUnits=N/m  PzDampingCoefficient=0  PzDampingCoefficientUnits=N/(m/s)  PzTorqueActuationMode=ComputedTorque  PzMotionActuationMode=InputMotion  PzSensePosition=off  PzSenseVelocity=off  PzSenseAcceleration=off  PzSenseTorqueForce=off  PzSenseLowerLimitTorqueForce=off  PzSenseUpperLimitTorqueForce=off  PzLowerLimitSpecify=off  PzLowerLimitBound=-1  PzLowerLimitBoundUnits=m  PzLowerLimitStiffness=1e6  PzLowerLimitStiffnessUnits=N/m  PzLowerLimitDamping=1e3  PzLowerLimitDampingUnits=N/(m/s)  PzLowerLimitTransitionRegionWidth=1e-4  PzLowerLimitTransitionRegionWidthUnits=m  PzUpperLimitSpecify=off  PzUpperLimitBound=1  PzUpperLimitBoundUnits=m  PzUpperLimitStiffness=1e6  PzUpperLimitStiffnessUnits=N/m  PzUpperLimitDamping=1e3  PzUpperLimitDampingUnits=N/(m/s)  PzUpperLimitTransitionRegionWidth=1e-4  PzUpperLimitTransitionRegionWidthUnits=m  PzPositionTargetSpecify=off  PzPositionTargetPriority=High  PzPositionTargetValue=0  PzPositionTargetValueUnits=m  PzVelocityTargetSpecify=off  PzVelocityTargetPriority=High  PzVelocityTargetValue=0  PzVelocityTargetValueUnits=m/s
  Gain : Gain  Gain=-1
  Gain1 : Gain  Gain=-1
  Mechanism Configuration : sm_lib/Utilities/Mechanism Configuration  UniformGravity=Constant  GravityVector=[0 0 -9.81]  GravityVectorUnits=m/s^2  GravityUnits=m/s^2  LinearizationDelta=0.001  JointModeTransitionNonlinearIterations=2
  PS-Simulink Converter : nesl_utility/PS-Simulink Converter  PhysicalDomain=network_engine_domain  SubClassName=ps_output  LeftPortType=input  RightPortType=output  PseudoPeriodic=off  Frequencies=[]  Unit=inherit  AffineConversion=off
      settings: SourceProductBaseCode=PW,SS
  PS-Simulink Converter1 : nesl_utility/PS-Simulink Converter  PhysicalDomain=network_engine_domain  SubClassName=ps_output  LeftPortType=input  RightPortType=output  PseudoPeriodic=off  Frequencies=[]  Unit=inherit  AffineConversion=off
      settings: SourceProductBaseCode=PW,SS
  PS-Simulink Converter2 : nesl_utility/PS-Simulink Converter  PhysicalDomain=network_engine_domain  SubClassName=ps_output  LeftPortType=input  RightPortType=output  PseudoPeriodic=off  Frequencies=[]  Unit=inherit  AffineConversion=off
      settings: SourceProductBaseCode=PW,SS
  Rigid Transform1 : sm_lib/Frames and Transforms/Rigid Transform  TranslationMethod=Cartesian  TranslationStandardOffset=0  TranslationLengthUnit=m  TranslationStandardAxis=+Z  TranslationCartesianOffset=[0 0 .45]  TranslationROffset=0  TranslationROffsetUnits=m  TranslationZOffset=0  TranslationZOffsetUnits=m  TranslationThetaOffset=0  TranslationThetaOffsetUnits=deg  RotationMethod=None  RotationAngleUnits=deg  RotationStandardAxis=+Z  RotationAngle=0.0  RotationArbitraryAxis=[0 0 1]  FollAlignAxisA=+X  BaseAlignAxisA=+Y  FollAlignAxisB=+Y  BaseAlignAxisB=+Z  RotationSequenceAxes=FollowerAxes  RotationSequence=XYX  RotationSequenceAngles=[0 0 0]  RotationSequenceAnglesUnits=deg  RotationMatrix=[1 0 0; 0 1 0; 0 0 1]
  Rigid Transform2 : sm_lib/Frames and Transforms/Rigid Transform  TranslationMethod=Cartesian  TranslationStandardOffset=0  TranslationLengthUnit=m  TranslationStandardAxis=+Z  TranslationCartesianOffset=[0 0 -1]  TranslationROffset=0  TranslationROffsetUnits=m  TranslationZOffset=0  TranslationZOffsetUnits=m  TranslationThetaOffset=0  TranslationThetaOffsetUnits=deg  RotationMethod=None  RotationAngleUnits=deg  RotationStandardAxis=+Z  RotationAngle=0.0  RotationArbitraryAxis=[0 0 1]  FollAlignAxisA=+X  BaseAlignAxisA=+Y  FollAlignAxisB=+Y  BaseAlignAxisB=+Z  RotationSequenceAxes=FollowerAxes  RotationSequence=XYX  RotationSequenceAngles=[0 0 0]  RotationSequenceAnglesUnits=deg  RotationMatrix=[1 0 0; 0 1 0; 0 0 1]
  Simple Rocket : sm_lib/Body Elements/File Solid  ExtGeomFileName=Rocket.stl  UnitType=Custom  ExtGeomFileUnits=m  StepReaderType=HEX  ExportConvexHullGeometry=off  InertiaType=Custom  Mass=0.8  MassUnits=kg  CenterOfMass=[0 0 .45]  CenterOfMassUnits=m  MomentsOfInertia=[1 1 1]  MomentsOfInertiaUnits=kg*m^2  ProductsOfInertia=[0 0 0]  ProductsOfInertiaUnits=kg*m^2  BasedOnType=Mass  Density=1000  DensityUnits=kg/m^3  DoExposeReferenceFrame=on  SerializedFrames=<Frames/>  GraphicType=FromGeometry  MarkerShape=Sphere  MarkerSize=10  GraphicVisPropType=SimpleVisualProperties  GraphicDiffuseColor=[1.0 0.4 0.0]  GraphicSpecularColor=[0.5 0.5 0.5 1.0]  GraphicAmbientColor=[0.15 0.15 0.15 1.0]  GraphicEmissiveColor=[0.0 0.0 0.0 1.0]  GraphicShininess=75  GraphicOpacity=1.0
  Simulink-PS Converter : nesl_utility/Simulink-PS Converter  PhysicalDomain=network_engine_domain  SubClassName=ps_input  LeftPortType=input  RightPortType=output  PseudoPeriodic=off  Frequencies=[]  NoiseDistribution=none  NoiseParameters=[]  Unit=1  AffineConversion=off  FilteringAndDerivatives=provide  SimscapeFilterOrder=1  InputFilterTimeConstant=0.001  UdotUserProvided=0
      settings: SourceProductBaseCode=PW,SS
  Simulink-PS Converter1 : nesl_utility/Simulink-PS Converter  PhysicalDomain=network_engine_domain  SubClassName=ps_input  LeftPortType=input  RightPortType=output  PseudoPeriodic=off  Frequencies=[]  NoiseDistribution=none  NoiseParameters=[]  Unit=1  AffineConversion=off  FilteringAndDerivatives=provide  SimscapeFilterOrder=1  InputFilterTimeConstant=0.001  UdotUserProvided=0
      settings: SourceProductBaseCode=PW,SS
  Simulink-PS Converter2 : nesl_utility/Simulink-PS Converter  PhysicalDomain=network_engine_domain  SubClassName=ps_input  LeftPortType=input  RightPortType=output  PseudoPeriodic=off  Frequencies=[]  NoiseDistribution=none  NoiseParameters=[]  Unit=1  AffineConversion=off  FilteringAndDerivatives=filter  SimscapeFilterOrder=2  InputFilterTimeConstant=0.01  UdotUserProvided=0
      settings: SourceProductBaseCode=PW,SS
  Simulink-PS Converter3 : nesl_utility/Simulink-PS Converter  PhysicalDomain=network_engine_domain  SubClassName=ps_input  LeftPortType=input  RightPortType=output  PseudoPeriodic=off  Frequencies=[]  NoiseDistribution=none  NoiseParameters=[]  Unit=1  AffineConversion=off  FilteringAndDerivatives=filter  SimscapeFilterOrder=2  InputFilterTimeConstant=0.01  UdotUserProvided=0
      settings: SourceProductBaseCode=PW,SS
  Simulink-PS Converter4 : nesl_utility/Simulink-PS Converter  PhysicalDomain=network_engine_domain  SubClassName=ps_input  LeftPortType=input  RightPortType=output  PseudoPeriodic=off  Frequencies=[]  NoiseDistribution=none  NoiseParameters=[]  Unit=1  AffineConversion=off  FilteringAndDerivatives=filter  SimscapeFilterOrder=2  InputFilterTimeConstant=0.01  UdotUserProvided=0
      settings: SourceProductBaseCode=PW,SS
  Simulink-PS Converter7 : nesl_utility/Simulink-PS Converter  PhysicalDomain=network_engine_domain  SubClassName=ps_input  LeftPortType=input  RightPortType=output  PseudoPeriodic=off  Frequencies=[]  NoiseDistribution=none  NoiseParameters=[]  Unit=1  AffineConversion=off  FilteringAndDerivatives=provide  SimscapeFilterOrder=1  InputFilterTimeConstant=0.001  UdotUserProvided=0
      settings: SourceProductBaseCode=PW,SS
  Solver Configuration : nesl_utility/Solver Configuration  PhysicalDomain=network_engine_domain  SubClassName=solver  LeftPortType=input  RightPortType=generic  Tones=[]  Harmonics=[]  SimulateNoise=off  Profile=off  UseLocalSampling=off  EnableSwitchedLinearOptims=on  FrequencyDomain=off  UseCCode=off  RelTol=0.001  AbsTol=1e-06  MinStep=1e-09  ToWorkspace=off  RevertToSquareIcSolve=off  NumHomotopyIterations=100  PhasorMode=off  PhasorModeNumHarmonics=1  DoDC=off  ResidualTolerance=1e-09  UseLocalSolver=off  LocalSolverChoice=NE_BACKWARD_EULER_ADVANCER  LocalSolverSampleTime=0.001  DoFixedCost=off  MaxNonlinIter=3  MaxModeIter=2  ComputeImpulses=off  ImpulseIterations=2  LinearAlgebra=Sparse  EquationFormulation=NE_TIME_EF  DelaysMemoryBudget=1024  AutomaticFiltering=on  FilteringTimeConstant=0.001  PartitionStorageMethod=AS_NEEDED  PartitionMemoryBudget=1024  PartitionMethod=FAST
      settings: SourceProductBaseCode=PW,SS
  Subsystem : Subsystem
  Transport Delay : TransportDelay  DelayTime=0.01  BufferSize=100
  Transport Delay1 : TransportDelay  DelayTime=0.01  BufferSize=100
  Transport Delay2 : TransportDelay  DelayTime=0.01  BufferSize=100
  World Frame : sm_lib/Frames and Transforms/World Frame
  cam01 : sm_lib/Frames and Transforms/Rigid Transform  TranslationMethod=Cartesian  TranslationStandardOffset=0  TranslationLengthUnit=m  TranslationStandardAxis=+Z  TranslationCartesianOffset=[0 -5.5 1]  TranslationROffset=0  TranslationROffsetUnits=m  TranslationZOffset=0  TranslationZOffsetUnits=m  TranslationThetaOffset=0  TranslationThetaOffsetUnits=deg  RotationMethod=AlignedAxes  RotationAngleUnits=deg  RotationStandardAxis=+Z  RotationAngle=0.0  RotationArbitraryAxis=[0 0 1]  FollAlignAxisA=+X  BaseAlignAxisA=+Y  FollAlignAxisB=+Y  BaseAlignAxisB=+Z  RotationSequenceAxes=FollowerAxes  RotationSequence=XYX  RotationSequenceAngles=[0 0 0]  RotationSequenceAnglesUnits=deg  RotationMatrix=[1 0 0; 0 1 0; 0 0 1]
  cam02 : sm_lib/Frames and Transforms/Rigid Transform  TranslationMethod=Cartesian  TranslationStandardOffset=0  TranslationLengthUnit=m  TranslationStandardAxis=+Z  TranslationCartesianOffset=[0 0 3.5]  TranslationROffset=0  TranslationROffsetUnits=m  TranslationZOffset=0  TranslationZOffsetUnits=m  TranslationThetaOffset=0  TranslationThetaOffsetUnits=deg  RotationMethod=StandardAxis  RotationAngleUnits=deg  RotationStandardAxis=+X  RotationAngle=90  RotationArbitraryAxis=[0 0 1]  FollAlignAxisA=+X  BaseAlignAxisA=+Y  FollAlignAxisB=+Y  BaseAlignAxisB=+Z  RotationSequenceAxes=FollowerAxes  RotationSequence=XYX  RotationSequenceAngles=[0 0 0]  RotationSequenceAnglesUnits=deg  RotationMatrix=[1 0 0; 0 1 0; 0 0 1]
  sideTrack : sm_lib/Frames and Transforms/Reference Frame
      settings: SourceProductName=Multibody
  trackCam : sm_lib/Frames and Transforms/Reference Frame
      settings: SourceProductName=Multibody
  Px : Outport
  Pz : Outport  Port=2
  wires:
  PS-Simulink Converter/1 -> Px/1, Transport Delay2/1
  Fz/1 -> Gain1/1
  M/1 -> Simulink-PS Converter7/1
  PS-Simulink Converter1/1 -> Transport Delay1/1
  Transport Delay2/1 -> Simulink-PS Converter4/1
  Transport Delay/1 -> Simulink-PS Converter2/1
  Transport Delay1/1 -> Simulink-PS Converter3/1
  PS-Simulink Converter2/1 -> Pz/1, Transport Delay/1
  Fx/1 -> Gain/1
  Gain/1 -> Simulink-PS Converter/1
  Gain1/1 -> Simulink-PS Converter1/1
  connections:
  Simulink-PS Converter4/RConn1 -- Cartesian Joint/LConn2
  PS-Simulink Converter/LConn1 -- 6-DOF Joint/RConn2
  Rigid Transform1/RConn1 -- 6-DOF Joint/RConn1
  Rigid Transform2/LConn1 -- 6-DOF Joint/LConn1
  Simulink-PS Converter2/RConn1 -- Cartesian Joint/LConn4
  Simulink-PS Converter3/RConn1 -- Cartesian Joint/LConn3
  PS-Simulink Converter2/LConn1 -- 6-DOF Joint/RConn4
  Simulink-PS Converter/RConn1 -- 6-DOF Joint/LConn2
  PS-Simulink Converter1/LConn1 -- 6-DOF Joint/RConn3
  Simulink-PS Converter7/RConn1 -- 6-DOF Joint/LConn4
  Rigid Transform1/LConn1 -- Simple Rocket/RConn1
  Simulink-PS Converter1/RConn1 -- 6-DOF Joint/LConn3
  Cartesian Joint/LConn1 -- Solver Configuration/RConn1 -- World Frame/RConn1 -- Rigid Transform2/RConn1 -- Mechanism Configuration/RConn1 -- Subsystem/LConn1
  Cartesian Joint/RConn1 -- cam01/LConn1 -- cam02/LConn1
  cam01/RConn1 -- sideTrack/RConn1
  cam02/RConn1 -- trackCam/RConn1

== system Flight_Model_2020b_11_28_2020/Aerodynamics/CP Forces and Moments/AOA ==
  Beta : Inport
  AOA : Outport
  wires:
  Beta/1 -> AOA/1

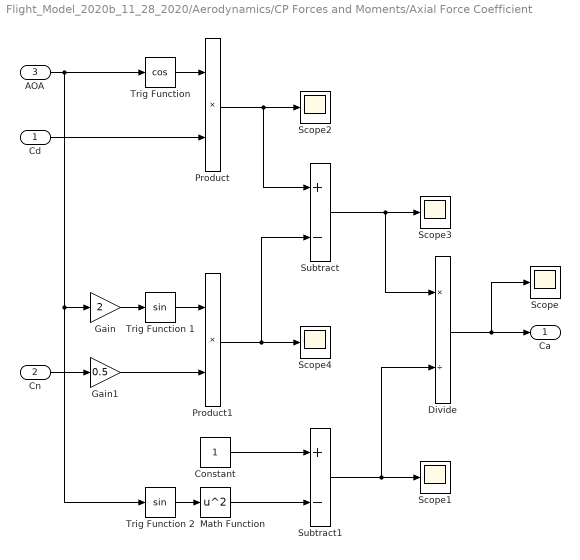
== system Flight_Model_2020b_11_28_2020/Aerodynamics/CP Forces and Moments/Axial Force Coefficient ==
  Cd : Inport
  Cn : Inport  Port=2
  AOA : Inport  Port=3
  Constant : Constant
  Divide : Product  Inputs=*/
  Gain : Gain  Gain=2
  Gain1 : Gain  Gain=0.5
  Math Function : Math  Operator=square  SignedPower=on  SaturateOnIntegerOverflow=on
  Product : Product
  Product1 : Product
  Scope{,1..4} (5 alike) : Scope
  Subtract : Sum  Inputs=+-
  Subtract1 : Sum  Inputs=+-
  Trig Function : Trigonometry  Operator=cos
  Trig Function 1 : Trigonometry
  Trig Function 2 : Trigonometry
  Ca : Outport
  wires:
  AOA/1 -> Trig Function/1, Trig Function 2/1, Gain/1
  Cd/1 -> Product/2
  Trig Function/1 -> Product/1
  Gain/1 -> Trig Function 1/1
  Trig Function 1/1 -> Product1/1
  Gain1/1 -> Product1/2
  Cn/1 -> Gain1/1
  Product1/1 -> Scope4/1, Subtract/2
  Divide/1 -> Scope/1, Ca/1
  Trig Function 2/1 -> Math Function/1
  Math Function/1 -> Subtract1/2
  Constant/1 -> Subtract1/1
  Subtract/1 -> Scope3/1, Divide/1
  Subtract1/1 -> Scope1/1, Divide/2
  Product/1 -> Scope2/1, Subtract/1

== system Flight_Model_2020b_11_28_2020/Aerodynamics/CP Forces and Moments/Axial Force Coefficient1 ==
  Cd : Inport
  AOA : Inport  Port=2
  Product : Product
  Scope : Scope
  Trig Function : Trigonometry  Operator=cos
  Ca : Outport
  wires:
  AOA/1 -> Trig Function/1
  Cd/1 -> Product/2
  Trig Function/1 -> Product/1
  Product/1 -> Ca/1, Scope/1

== system Flight_Model_2020b_11_28_2020/Aerodynamics/CP Forces and Moments/Axial Forces ==
  Ca : Inport
  Aref : Inport  Port=2
  "q " : Inport  Port=3
  Product : Product  Inputs=3
  Scope : Scope
  Axial Force : Outport
  wires:
  Ca/1 -> Product/1
  Aref/1 -> Product/2
  Product/1 -> Axial Force/1, Scope/1
  "q "/1 -> Product/3

== system Flight_Model_2020b_11_28_2020/Aerodynamics/CP Forces and Moments/Drag Force Coefficient ==
  In1 : Inport
  Cd : Outport
  wires:
  In1/1 -> Cd/1

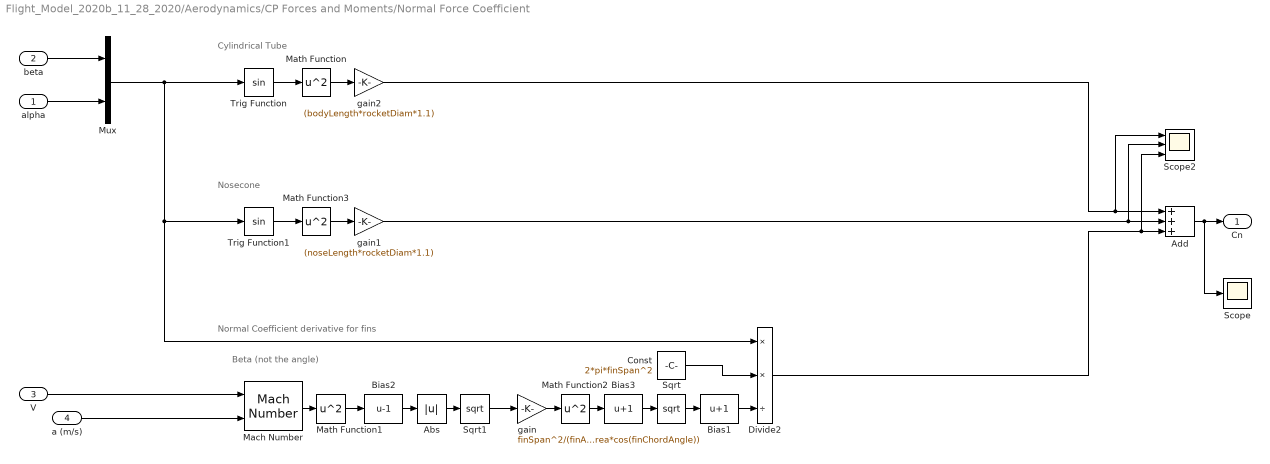
== system Flight_Model_2020b_11_28_2020/Aerodynamics/CP Forces and Moments/Normal Force Coefficient ==
  note: Cylindrical Tube
  note: Normal Coefficient derivative for fins
  note: Beta (not the angle)
  note: Nosecone
  alpha : Inport
  beta : Inport  Port=2
  V : Inport  Port=3
  a (m/s) : Inport  Port=4
  Abs : Abs
  Add : Sum  Inputs=+++
  Bias1 : Bias  Bias=1
  Bias2 : Bias  Bias=-1
  Bias3 : Bias  Bias=1
  Const : Constant  Value=2*pi*finSpan^2
  Divide2 : Product  Inputs=**/
  Mach Number : aerolibasang/Mach Number
      settings: SourceProductBaseCode=AE
  Math Function{,1..3} (4 alike) : Math  Operator=square  SignedPower=on  SaturateOnIntegerOverflow=on
  Mux : Mux  Inputs=2
  Scope : Scope
  Scope2 : Scope  NumInputPorts=3
  Sqrt : Sqrt  SaturateOnIntegerOverflow=on
  Sqrt1 : Sqrt  SaturateOnIntegerOverflow=on
  Trig Function : Trigonometry
  Trig Function1 : Trigonometry
  gain : Gain  Gain=finSpan^2/(finArea*cos(finChordAngle))
  gain1 : Gain  Gain=(noseLength*rocketDiam*1.1)
  gain2 : Gain  Gain=(bodyLength*rocketDiam*1.1)
  Cn : Outport
  wires:
  Trig Function/1 -> Math Function/1
  Sqrt1/1 -> gain/1
  Math Function2/1 -> Bias3/1
  Sqrt/1 -> Bias1/1
  Bias3/1 -> Sqrt/1
  gain/1 -> Math Function2/1
  a (m/s)/1 -> Mach Number/2
  Bias1/1 -> Divide2/3
  Math Function/1 -> gain2/1
  Trig Function1/1 -> Math Function3/1
  Math Function3/1 -> gain1/1
  Add/1 -> Scope/1, Cn/1
  V/1 -> Mach Number/1
  Mach Number/1 -> Math Function1/1
  Math Function1/1 -> Bias2/1
  Bias2/1 -> Abs/1
  Abs/1 -> Sqrt1/1
  Mux/1 -> Divide2/1, Trig Function1/1, Trig Function/1
  Const/1 -> Divide2/2
  gain1/1 -> Scope2/2, Add/2
  gain2/1 -> Add/1, Scope2/1
  Divide2/1 -> Add/3, Scope2/3
  alpha/1 -> Mux/2
  beta/1 -> Mux/1

== system Flight_Model_2020b_11_28_2020/Aerodynamics/CP Forces and Moments/Normal Forces ==
  Cn : Inport
  Aref : Inport  Port=2
  "q " : Inport  Port=3
  Product : Product  Inputs=3
  Scope : Scope
  Normal Force : Outport
  wires:
  Cn/1 -> Product/1
  Aref/1 -> Product/2
  Product/1 -> Normal Force/1, Scope/1
  "q "/1 -> Product/3

== system Flight_Model_2020b_11_28_2020/Avionics/Pressure Sensor/Pressure to Altitude ==
  note: \/ \/ to power of 1/5.257
  note: presser & temp to altitude
  Atmostpheric Pressure : Inport
  "Temp (C) " : Inport  Port=2
  Add : Sum
  Constant : Constant  Value=273.15
  Constant1 : Constant  Value=.0065
  Constant2 : Constant
  Divide : Product  Inputs=*/
  Divide1 : Product  Inputs=*/
  Fcn : Fcn  Expr=u^0.19022256039
  Product : Product
  Subtract : Sum  Inputs=+-
  sealevel pressure : Constant  Value=1013.25
  Altitude : Outport
  wires:
  Constant/1 -> Add/2
  "Temp (C) "/1 -> Add/1
  Constant1/1 -> Divide/2
  Constant2/1 -> Subtract/2
  Add/1 -> Product/2
  Atmostpheric Pressure/1 -> Divide1/2
  sealevel pressure/1 -> Divide1/1
  Divide/1 -> Altitude/1
  Subtract/1 -> Product/1
  Product/1 -> Divide/1
  Fcn/1 -> Subtract/1
  Divide1/1 -> Fcn/1
